simulink model "simulinkFrame"  (R2017a)
settings: Solver=VariableStepAuto  StartTime=0.0  StopTime=tEnd  FixedStep=0.01  MaxStep=1e-2  RelTol=1e-3  EnableMultiTasking=on
undefined symbols (not defined in the file or in its folder): bf, Dtheta0, sampleTime, theta0
libraries: simulink x2
settings Model: Creator=christfs  LastModifiedBy=christfs
settings DataIOCC: LimitDataPoints=on
settings OptimizationCC: LifeSpan=inf
settings DebuggingCC: AllowSymbolicDim=off  SFUnexpectedBacktrackingDiag=warning  SFNoUnconditionalDefaultTransitionDiag=warning  SFExecutionAtInitializationDiag=none
settings ModelReferenceCC: PropagateSignalLabelsOutOfModel=off
settings GRTTargetCC: TargetLangStandard=C89/C90 (ANSI)
settings ConfigComp: CovMetricSettings=dw  CovHtmlReporting=on  CovSaveCumulativeToWorkspaceVar=on  CovSaveSingleToWorkspaceVar=on  CovExternalEMLEnable=off

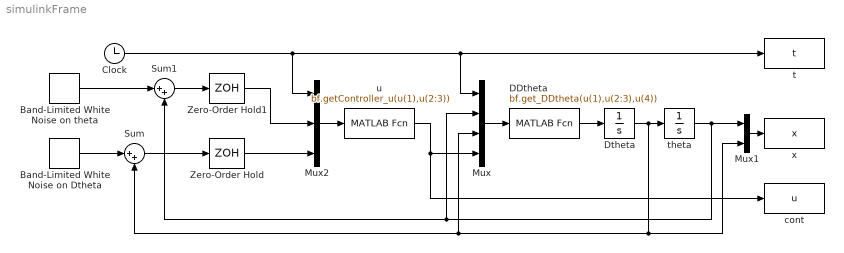
== system simulinkFrame ==
  " DDtheta" : MATLABFcn  MATLABFcn=bf.get_DDtheta(u(1),u(2:3),u(4))
  Band-Limited White Noise on Dtheta : simulink/Sources/Band-Limited White Noise  Cov=noisepw  Ts=sampleTime  seed=[23342]
  Band-Limited White Noise on theta : simulink/Sources/Band-Limited White Noise  Cov=noisepw  Ts=sampleTime  seed=[23341]
  Clock : Clock
  Dtheta : Integrator  InitialCondition=Dtheta0
  Mux : Mux
  Mux1 : Mux  Inputs=2
  Mux2 : Mux  Inputs=3
  Sum : Sum  Inputs=|++
  Sum1 : Sum  Inputs=|++
  Zero-Order Hold : ZeroOrderHold  SampleTime=-1
  Zero-Order Hold1 : ZeroOrderHold  SampleTime=-1
  cont : ToWorkspace  VariableName=u  SampleTime=-1
  t : ToWorkspace  VariableName=t  SampleTime=-1
  theta : Integrator  InitialCondition=theta0
  u : MATLABFcn  MATLABFcn=bf.getController_u(u(1),u(2:3))
  x : ToWorkspace  VariableName=x  SampleTime=-1
  wires:
  Clock/1 -> Mux/1, t/1, Mux2/1
  " DDtheta"/1 -> Dtheta/1
  Mux1/1 -> x/1
  Mux/1 -> " DDtheta"/1
  Band-Limited White Noise on Dtheta/1 -> Sum/1
  Dtheta/1 -> theta/1, Mux1/2, Sum/2, Mux/3
  theta/1 -> Mux1/1, Mux/2, Sum1/2
  Sum1/1 -> Zero-Order Hold1/1
  Sum/1 -> Zero-Order Hold/1
  Mux2/1 -> u/1
  u/1 -> cont/1, Mux/4
  Zero-Order Hold/1 -> Mux2/3
  Zero-Order Hold1/1 -> Mux2/2
  Band-Limited White Noise on theta/1 -> Sum1/1
